simulink model "aliasing_demo"  (Simulink 10.1)
settings: Solver=ode45  StartTime=0.0  StopTime=5  RelTol=1e-3  EnableMultiTasking=on
settings Model: Creator=rcheng  LastModifiedBy=juan
settings DataIOCC: LimitDataPoints=on  SignalLoggingSaveFormat=ModelDataLogs
settings OptimizationCC: ExpressionDepthLimit=2147483647  InitFltsAndDblsToZero=on
settings DebuggingCC: SolverPrmCheckMsg=warning  FcnCallInpInsideContextMsg=warning  StateNameClashWarn=warning
settings ConfigComp: CovHtmlReporting=off  CovSFcnEnable=off

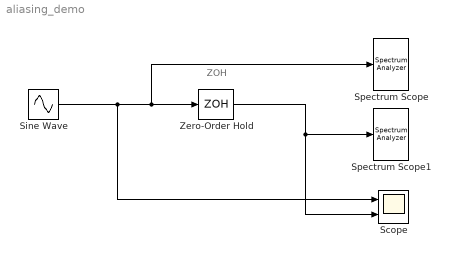
== system aliasing_demo ==
  note: ZOH
  Scope : Scope  NumInputPorts=2
  Sine Wave : Sin  Amplitude=5  Frequency=2*pi*100  SampleTime=1/10000
  Spectrum Scope : SpectrumAnalyzer
  Spectrum Scope1 : SpectrumAnalyzer
  Zero-Order Hold : ZeroOrderHold  SampleTime=1/1000
  wires:
  Zero-Order Hold/1 -> Spectrum Scope1/1, Scope/2
  Sine Wave/1 -> Scope/1, Spectrum Scope/1, Zero-Order Hold/1
